simulink model "advisor_ess_options"  (Simulink 2.20)
settings: Solver=ode1  StartTime=0.0  StopTime=500  FixedStep=1  RelTol=1e-3
values from neighbouring files (symbols this model uses):
  amb_tmp = vinf.test.ambtmp    [RW_execute.m]
  cyc_mph = [time speed]    [DataCompareFigControl.m]    (also in J17_FUDS.m = [time_vec speed_vec]; J17_HFEDS.m = [time_vec speed_vec]; J17_SC03.m = [time_vec speed_vec]; J17_UDDS.m = [time_vec speed_vec])
  ess_init_soc = vinf.test.ess_init_soc.FUDS    [J17_FUDS.m]    (also in J17_HFEDS.m = vinf.test.ess_init_soc.HWFET; J17_SC03.m = vinf.test.ess_init_soc.SC03; J17_UDDS.m = vinf.test.ess_init_soc.UDDS; J17_US06.m = vinf.test.ess_init_soc.US06)
undefined symbols (not defined in the file or in its folder): air_cp, enable_stop, ess_coulombic_eff, ess_max_ah_cap, ess_max_p, ess_max_p_soc, ess_max_volts, ess_min_volts, ess_MMi, ess_MMo, ess_mod_airflow, ess_mod_cp, ess_mod_init_tmp, ess_module_mass, ess_module_num, ess_on, ess_set_tmp, ess_th_calc, ess_th_res_off, ess_th_res_on, ess_tmp, fund_byu, fund_byuop, mc_min_volts, t_soc
(part 1 of 2)
settings Model: ConsistencyChecking=off  RTWPlaceOutputsASAP=off

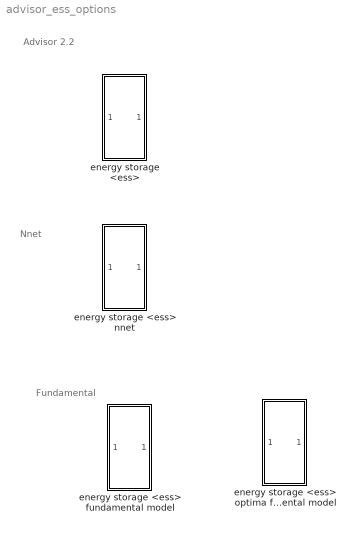
== system advisor_ess_options ==
  note: Nnet
  note: Fundamental
  note: Advisor 2.2
  energy storage <ess> : Subsystem
  energy storage <ess> nnet : Subsystem
  energy storage <ess> fundamental model : Subsystem
  energy storage <ess> optima fundamental model : Subsystem

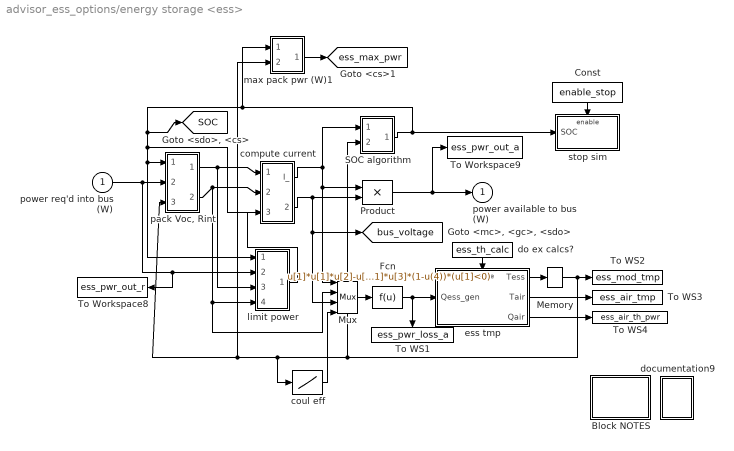
== system advisor_ess_options/energy storage <ess> ==
  power req'd into bus (W) : Inport  Port=1  PortWidth=-1  SampleTime=-1
  Block NOTES : Subsystem
      mask Display: disp('Block\nNOTES')
  Const : Constant  Orientation=down  Value=enable_stop
  Fcn : Fcn  Expr=u[1]*u[1]*u[2]-u[1]*u[3]*(1-u(4))*(u[1]<0)
  Memory : Memory  X0=amb_tmp  InheritSampleTime=off
  Mux : Mux  Inputs=4
  Product : Product  Inputs=2
  SOC algorithm : Subsystem
  To WS1 : ToWorkspace  VariableName=ess_pwr_loss_a  SampleTime=0
      settings: Orientation=down
  To WS2 : ToWorkspace  VariableName=ess_mod_tmp  SampleTime=0
  To WS3 : ToWorkspace  VariableName=ess_air_tmp  SampleTime=0
  To WS4 : ToWorkspace  VariableName=ess_air_th_pwr  SampleTime=0
  To Workspace8 : ToWorkspace  VariableName=ess_pwr_out_r  SampleTime=-1
  To Workspace9 : ToWorkspace  VariableName=ess_pwr_out_a  SampleTime=-1
  compute current : Subsystem
  coul eff : Lookup  InputValues=ess_tmp  OutputValues=ess_coulombic_eff
  do ex calcs? : Constant  Orientation=down  Value=ess_th_calc
  documentation9 : Subsystem
      settings: OpenFcn=web(['file:\\\' which('energy_storage.htm')]);
      mask Display: image(imread('doc_man.jpg'))
  ess tmp : Subsystem
  limit power : Subsystem
  max pack pwr (W)1 : Subsystem
  "pack Voc, Rint" : Subsystem
  stop sim : Subsystem
  power available to bus (W) : Outport  Port=1  InitialOutput=0
  tag scope: SOC=global, bus_voltage=global, ess_max_pwr=global
  wires:
  Memory/1 -> max pack pwr (W)1/2(ess_mod_tmp), "pack Voc, Rint"/3(mod tmp   (C)), coul eff/1, SOC algorithm/2(tmp (C)), To WS2/1
  max pack pwr (W)1/1(max ess discharge pwr) -> [ess_max_pwr]
  coul eff/1 -> Mux/4
  ess tmp/1(Tess) -> Memory/1
  ess tmp/3(Qair) -> To WS4/1
  ess tmp/2(Tair) -> To WS3/1
  limit power/1("Pbty, limited") -> compute current/3(limited output power (W))
  "pack Voc, Rint"/1(pack open- circuit voltage) -> limit power/3(Voc), compute current/1(Voc)
  "pack Voc, Rint"/2(pack resistance) -> Mux/2, limit power/4(Rint), compute current/2(Rint)
  Const/1 -> stop sim/Enable
  SOC algorithm/1(SOC1) -> max pack pwr (W)1/1(SOC), limit power/1(SOC), "pack Voc, Rint"/1(SOC (prev)), [SOC], stop sim/1(SOC)
  do ex calcs?/1 -> ess tmp/Enable
  Fcn/1 -> ess tmp/1(Qess_gen), To WS1/1
  Product/1 -> power available to bus (W)/1, To Workspace9/1
  compute current/1(I_) -> Mux/1, Product/1, SOC algorithm/1((A))
  power req'd into bus (W)/1 -> "pack Voc, Rint"/2(req'd battery power (W)), limit power/2(Pbty), To Workspace8/1
  Mux/1 -> Fcn/1
  compute current/2(V_) -> [bus_voltage], Mux/3, Product/2

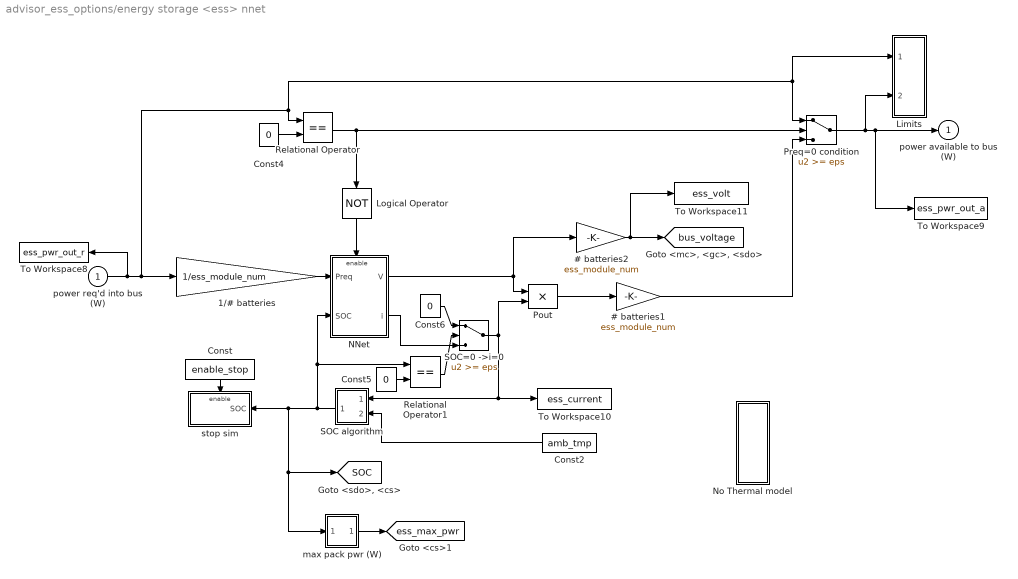
== system advisor_ess_options/energy storage <ess> nnet ==
  power req'd into bus (W) : Inport  Port=1  PortWidth=-1  SampleTime=-1
  # batteries1 : Gain  Gain=ess_module_num
  # batteries2 : Gain  Gain=ess_module_num
  1/# batteries : Gain  Gain=1/ess_module_num
  Const : Constant  Orientation=down  Value=enable_stop
  Const2 : Constant  Orientation=left  Value=amb_tmp
  Const4 : Constant  Value=0
  Const5 : Constant  Value=0
  Const6 : Constant  Value=0
  Limits : Subsystem
  Logical Operator : Logic  Orientation=down  Operator=NOT  Inputs=1
  NNet : Subsystem
  No Thermal model : Subsystem
  Pout : Product  Inputs=2
  Preq=0 condition : Switch  Threshold=eps
  Relational Operator : RelationalOperator  Operator===
  Relational Operator1 : RelationalOperator  Operator===
  SOC algorithm : Subsystem  Orientation=left
  SOC=0 ->i=0 : Switch  Threshold=eps
  To Workspace10 : ToWorkspace  VariableName=ess_current  SampleTime=-1
  To Workspace11 : ToWorkspace  VariableName=ess_volt  SampleTime=-1
  To Workspace8 : ToWorkspace  VariableName=ess_pwr_out_r  SampleTime=-1
  To Workspace9 : ToWorkspace  VariableName=ess_pwr_out_a  SampleTime=-1
  max pack pwr (W) : Subsystem
  stop sim : Subsystem  Orientation=left
  power available to bus (W) : Outport  Port=1  InitialOutput=0
  tag scope: SOC=global, bus_voltage=global, ess_max_pwr=global
  wires:
  Const/1 -> stop sim/Enable
  SOC algorithm/1(SOC1) -> stop sim/1(SOC), [SOC], max pack pwr (W)/1(SOC), NNet/2(SOC), Relational Operator1/1
  power req'd into bus (W)/1 -> To Workspace8/1, 1/# batteries/1, Relational Operator/1, Preq=0 condition/1, Limits/1(power req)
  1/# batteries/1 -> NNet/1(Preq)
  Const4/1 -> Relational Operator/2
  Logical Operator/1 -> NNet/Enable
  Relational Operator/1 -> Preq=0 condition/2, Logical Operator/1
  max pack pwr (W)/1(ess discharge pwr) -> [ess_max_pwr]
  Pout/1 -> # batteries1/1
  NNet/1(V) -> Pout/1, # batteries2/1
  # batteries2/1 -> [bus_voltage], To Workspace11/1
  # batteries1/1 -> Preq=0 condition/3
  Preq=0 condition/1 -> power available to bus (W)/1, To Workspace9/1, Limits/2(power  available from battery)
  Const2/1 -> SOC algorithm/2(tmp (C))
  Const6/1 -> SOC=0 ->i=0/1
  NNet/2(i) -> SOC=0 ->i=0/3
  Const5/1 -> Relational Operator1/2
  Relational Operator1/1 -> SOC=0 ->i=0/2
  SOC=0 ->i=0/1 -> SOC algorithm/1((A)), To Workspace10/1, Pout/2

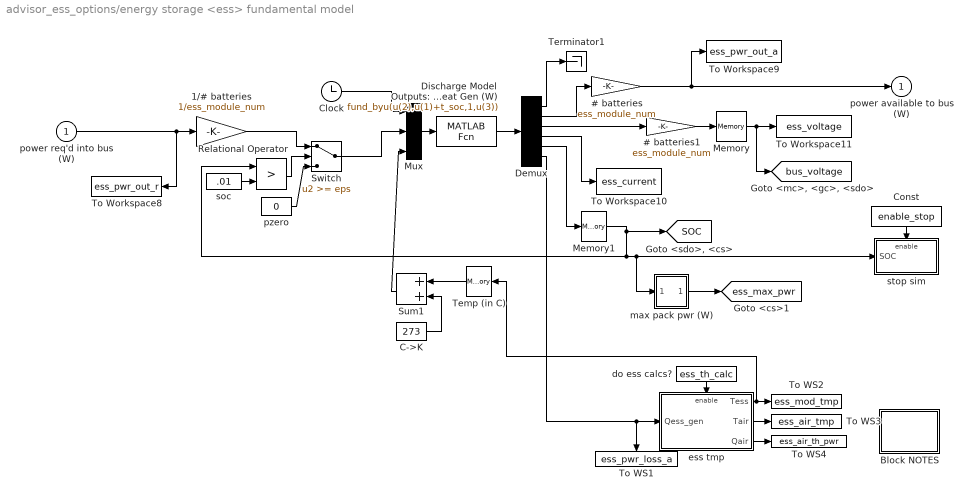
== system advisor_ess_options/energy storage <ess> fundamental model ==
  power req'd into bus (W) : Inport  Port=1  PortWidth=-1  SampleTime=-1
  # batteries : Gain  Gain=ess_module_num
  # batteries1 : Gain  Gain=ess_module_num
  1/# batteries : Gain  Gain=1/ess_module_num
  Block NOTES : Subsystem
      mask Display: disp('Block\nNOTES')
  C->K : Constant  Value=273
  Clock : Clock
  Const : Constant  Orientation=down  Value=enable_stop
  Demux : Demux  Outputs=6
  Discharge Model Outputs: Preq(W) Pavail (W) Voltage (V) Current (A) SOC Heat Gen (W) : MATLABFcn  MATLABFcn=fund_byu(u(2),u(1)+t_soc,1,u(3))  OutputWidth=-1
  Memory : Memory  X0=12*ess_module_num  InheritSampleTime=off
  Memory1 : Memory  X0=ess_init_soc  InheritSampleTime=off
  Mux : Mux  Inputs=3
  Relational Operator : RelationalOperator  Operator=>
  Sum1 : Sum  Orientation=left  Inputs=++
  Switch : Switch  Threshold=eps
  Temp (in C) : Memory  Orientation=left  X0=amb_tmp  InheritSampleTime=off
  Terminator1 : Terminator
  To WS1 : ToWorkspace  VariableName=ess_pwr_loss_a  SampleTime=0
      settings: Orientation=down  Buffer=50000
  To WS2 : ToWorkspace  VariableName=ess_mod_tmp  SampleTime=0
      settings: Buffer=50000
  To WS3 : ToWorkspace  VariableName=ess_air_tmp  SampleTime=0
      settings: Buffer=50000
  To WS4 : ToWorkspace  VariableName=ess_air_th_pwr  SampleTime=0
      settings: Buffer=50000
  To Workspace10 : ToWorkspace  VariableName=ess_current  SampleTime=-1
  To Workspace11 : ToWorkspace  VariableName=ess_voltage  SampleTime=-1
  To Workspace8 : ToWorkspace  VariableName=ess_pwr_out_r  SampleTime=-1
  To Workspace9 : ToWorkspace  VariableName=ess_pwr_out_a  SampleTime=-1
  do ess calcs? : Constant  Orientation=down  Value=ess_th_calc
  ess tmp : Subsystem
  max pack pwr (W) : Subsystem
  pzero : Constant  Value=0
  soc : Constant  Value=.01
  stop sim : Subsystem
  power available to bus (W) : Outport  Port=1  InitialOutput=0
  tag scope: SOC=global, bus_voltage=global, ess_max_pwr=global
  wires:
  Mux/1 -> Discharge Model Outputs: Preq(W) Pavail (W) Voltage (V) Current (A) SOC Heat Gen (W)/1
  Discharge Model Outputs: Preq(W) Pavail (W) Voltage (V) Current (A) SOC Heat Gen (W)/1 -> Demux/1
  Demux/5 -> Memory1/1
  Demux/4 -> To Workspace10/1
  Demux/2 -> # batteries/1
  Clock/1 -> Mux/1
  power req'd into bus (W)/1 -> To Workspace8/1, 1/# batteries/1
  pzero/1 -> Switch/3
  Relational Operator/1 -> Switch/2
  soc/1 -> Relational Operator/2
  1/# batteries/1 -> Switch/1
  Switch/1 -> Mux/2
  Demux/1 -> Terminator1/1
  # batteries/1 -> To Workspace9/1, power available to bus (W)/1
  # batteries1/1 -> Memory/1
  Demux/3 -> # batteries1/1
  Memory/1 -> To Workspace11/1, [bus_voltage]
  Memory1/1 -> Relational Operator/1, stop sim/1(SOC), max pack pwr (W)/1(SOC), [SOC]
  Temp (in C)/1 -> Sum1/1
  C->K/1 -> Sum1/2
  Sum1/1 -> Mux/3
  Const/1 -> stop sim/Enable
  max pack pwr (W)/1(ess discharge pwr) -> [ess_max_pwr]
  Demux/6 -> ess tmp/1(Qess_gen), To WS1/1
  do ess calcs?/1 -> ess tmp/Enable
  ess tmp/2(Tair) -> To WS3/1
  ess tmp/3(Qair) -> To WS4/1
  ess tmp/1(Tess) -> To WS2/1, Temp (in C)/1

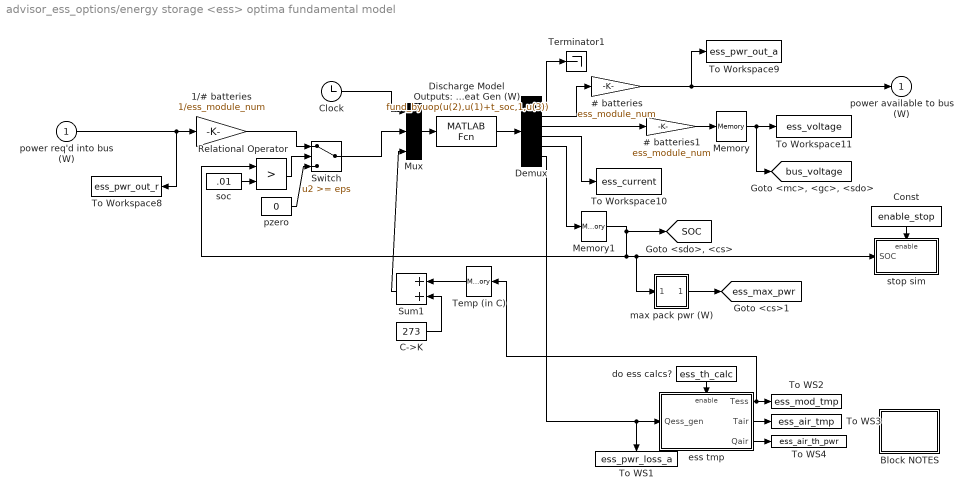
== system advisor_ess_options/energy storage <ess> optima fundamental model ==
  power req'd into bus (W) : Inport  Port=1  PortWidth=-1  SampleTime=-1
  # batteries : Gain  Gain=ess_module_num
  # batteries1 : Gain  Gain=ess_module_num
  1/# batteries : Gain  Gain=1/ess_module_num
  Block NOTES : Subsystem
      mask Display: disp('Block\nNOTES')
  C->K : Constant  Value=273
  Clock : Clock
  Const : Constant  Orientation=down  Value=enable_stop
  Demux : Demux  Outputs=6
  Discharge Model Outputs: Preq(W) Pavail (W) Voltage (V) Current (A) SOC Heat Gen (W) : MATLABFcn  MATLABFcn=fund_byuop(u(2),u(1)+t_soc,1,u(3))  OutputWidth=-1
  Memory : Memory  X0=12*ess_module_num  InheritSampleTime=off
  Memory1 : Memory  X0=ess_init_soc  InheritSampleTime=off
  Mux : Mux  Inputs=3
  Relational Operator : RelationalOperator  Operator=>
  Sum1 : Sum  Orientation=left  Inputs=++
  Switch : Switch  Threshold=eps
  Temp (in C) : Memory  Orientation=left  X0=amb_tmp  InheritSampleTime=off
  Terminator1 : Terminator
  To WS1 : ToWorkspace  VariableName=ess_pwr_loss_a  SampleTime=0
      settings: Orientation=down  Buffer=50000
  To WS2 : ToWorkspace  VariableName=ess_mod_tmp  SampleTime=0
      settings: Buffer=50000
  To WS3 : ToWorkspace  VariableName=ess_air_tmp  SampleTime=0
      settings: Buffer=50000
  To WS4 : ToWorkspace  VariableName=ess_air_th_pwr  SampleTime=0
      settings: Buffer=50000
  To Workspace10 : ToWorkspace  VariableName=ess_current  SampleTime=-1
  To Workspace11 : ToWorkspace  VariableName=ess_voltage  SampleTime=-1
  To Workspace8 : ToWorkspace  VariableName=ess_pwr_out_r  SampleTime=-1
  To Workspace9 : ToWorkspace  VariableName=ess_pwr_out_a  SampleTime=-1
  do ess calcs? : Constant  Orientation=down  Value=ess_th_calc
  ess tmp : Subsystem
  max pack pwr (W) : Subsystem
  pzero : Constant  Value=0
  soc : Constant  Value=.01
  stop sim : Subsystem
  power available to bus (W) : Outport  Port=1  InitialOutput=0
  tag scope: SOC=global, bus_voltage=global, ess_max_pwr=global
  wires:
  Mux/1 -> Discharge Model Outputs: Preq(W) Pavail (W) Voltage (V) Current (A) SOC Heat Gen (W)/1
  Discharge Model Outputs: Preq(W) Pavail (W) Voltage (V) Current (A) SOC Heat Gen (W)/1 -> Demux/1
  Demux/5 -> Memory1/1
  Demux/4 -> To Workspace10/1
  Demux/2 -> # batteries/1
  Clock/1 -> Mux/1
  power req'd into bus (W)/1 -> To Workspace8/1, 1/# batteries/1
  pzero/1 -> Switch/3
  Relational Operator/1 -> Switch/2
  soc/1 -> Relational Operator/2
  1/# batteries/1 -> Switch/1
  Switch/1 -> Mux/2
  Demux/1 -> Terminator1/1
  # batteries/1 -> To Workspace9/1, power available to bus (W)/1
  # batteries1/1 -> Memory/1
  Demux/3 -> # batteries1/1
  Memory/1 -> To Workspace11/1, [bus_voltage]
  Memory1/1 -> Relational Operator/1, stop sim/1(SOC), max pack pwr (W)/1(SOC), [SOC]
  Temp (in C)/1 -> Sum1/1
  C->K/1 -> Sum1/2
  Sum1/1 -> Mux/3
  Const/1 -> stop sim/Enable
  max pack pwr (W)/1(ess discharge pwr) -> [ess_max_pwr]
  Demux/6 -> ess tmp/1(Qess_gen), To WS1/1
  do ess calcs?/1 -> ess tmp/Enable
  ess tmp/2(Tair) -> To WS3/1
  ess tmp/3(Qair) -> To WS4/1
  ess tmp/1(Tess) -> To WS2/1, Temp (in C)/1

== system advisor_ess_options/energy storage <ess>/Block NOTES ==
  note: This block models the energy storage system as an SOC-dependent voltage
      | in series with an SOC- and current direction-dependent internal resistance.
      | SOC is computed assuming that A-h capacity is constant, but limited
      | such that a minimum voltage is never exceeded (replacing the
      | previous Peukert relationship which underpredicted battery capacity).
      |
      | Discharge power is limited here so as not to bring the bus (battery pack) voltage below
      | the minimum controller voltage or the minimum battery voltage and so as to allow
      | the solution of the quadratic eq'n for discharge current.
      |
      | Charge current is limited to ensure the voltage does not exceed a maximum
      | voltage
      |
      | Positive current is discharge current in the convention used here.
      | Power loss is computed as I*R+losses due to Coulombic (in)efficiency.
      |
      | Thermal modeling of the battery performance is modeled in the
      | OCV, Rint, and capacity.

== system advisor_ess_options/energy storage <ess>/SOC algorithm ==
  note: SOC=(Max Ah capacity-Ah used)/Max Ah capacity
  (A) : Inport  Port=1  PortWidth=-1  SampleTime=-1
  tmp (C) : Inport  Port=2  PortWidth=-1  SampleTime=-1
  (sec->hrs) : Gain  Gain=1/3600
  0 <= SOC <= 1 : Saturate  UpperLimit=1  LowerLimit=0
  A-h remaining : Sum  Inputs=-+
  Ah used : Integrator  ExternalReset=none  InitialConditionSource=external  InitialCondition=(1-ess_init_soc)*ess_max_ah_cap  LimitOutput=off  UpperSaturationLimit=inf  LowerSaturationLimit=-inf  ShowSaturationPort=off  ShowStatePort=off  AbsoluteTolerance=auto
  Fcn : Fcn  Expr=1/u
  Fcn1 : Fcn  Expr=(1-ess_init_soc)*u
  SOC : Product  Inputs=2
  Switch : Switch  Threshold=0
  adjusted A : Product  Inputs=2
  coul eff : Lookup  InputValues=ess_tmp  OutputValues=ess_coulombic_eff
  max cap : Lookup  InputValues=ess_tmp  OutputValues=ess_max_ah_cap
  SOC1 : Outport  Port=1  InitialOutput=0
  wires:
  Fcn1/1 -> Ah used/2
  max cap/1 -> Fcn1/1, Fcn/1, A-h remaining/2
  adjusted A/1 -> Switch/3
  coul eff/1 -> adjusted A/2
  tmp (C)/1 -> coul eff/1, max cap/1
  0 <= SOC <= 1/1 -> SOC1/1
  A-h remaining/1 -> SOC/1
  SOC/1 -> 0 <= SOC <= 1/1
  Fcn/1 -> SOC/2
  Ah used/1 -> A-h remaining/1
  (sec->hrs)/1 -> Ah used/1
  Switch/1 -> (sec->hrs)/1
  (A)/1 -> adjusted A/1, Switch/1, Switch/2

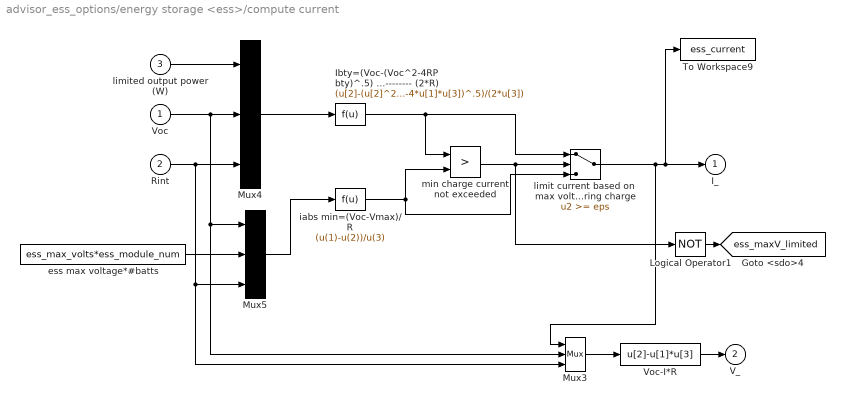
== system advisor_ess_options/energy storage <ess>/compute current ==
  Voc : Inport  Port=1  PortWidth=-1  SampleTime=-1
  Rint : Inport  Port=2  PortWidth=-1  SampleTime=-1
  limited output power (W) : Inport  Port=3  PortWidth=-1  SampleTime=-1
  Ibty=(Voc-(Voc^2-4RPbty)^.5)        ----------------------------- (2*R) : Fcn  Expr=(u[2]-(u[2]^2-4*u[1]*u[3])^.5)/(2*u[3])
  Logical Operator1 : Logic  Operator=NOT  Inputs=1
  Mux3 : Mux  Inputs=3
  Mux4 : Mux  Inputs=3
  Mux5 : Mux  Inputs=3
  To Workspace9 : ToWorkspace  VariableName=ess_current  SampleTime=-1
  Voc-I*R : Fcn  Expr=u[2]-u[1]*u[3]
  ess max voltage*#batts : Constant  Value=ess_max_volts*ess_module_num
  iabs min=(Voc-Vmax)/R : Fcn  Expr=(u(1)-u(2))/u(3)
  limit current based on  max voltage during charge : Switch  Threshold=eps
  min charge current not exceeded : RelationalOperator  Operator=>
  I_ : Outport  Port=1  InitialOutput=0
  V_ : Outport  Port=2  InitialOutput=0
  tag scope: ess_maxV_limited=global
  wires:
  Logical Operator1/1 -> [ess_maxV_limited]
  ess max voltage*#batts/1 -> Mux5/2
  Mux5/1 -> iabs min=(Voc-Vmax)/R/1
  Mux4/1 -> Ibty=(Voc-(Voc^2-4RPbty)^.5)        ----------------------------- (2*R)/1
  Voc-I*R/1 -> V_/1
  Mux3/1 -> Voc-I*R/1
  min charge current not exceeded/1 -> Logical Operator1/1, limit current based on  max voltage during charge/2
  limit current based on  max voltage during charge/1 -> Mux3/1, To Workspace9/1, I_/1
  iabs min=(Voc-Vmax)/R/1 -> limit current based on  max voltage during charge/3, min charge current not exceeded/2
  Ibty=(Voc-(Voc^2-4RPbty)^.5)        ----------------------------- (2*R)/1 -> limit current based on  max voltage during charge/1, min charge current not exceeded/1
  Rint/1 -> Mux5/3, Mux3/3, Mux4/3
  Voc/1 -> Mux5/1, Mux3/2, Mux4/2
  limited output power (W)/1 -> Mux4/1

== system advisor_ess_options/energy storage <ess>/documentation9 ==

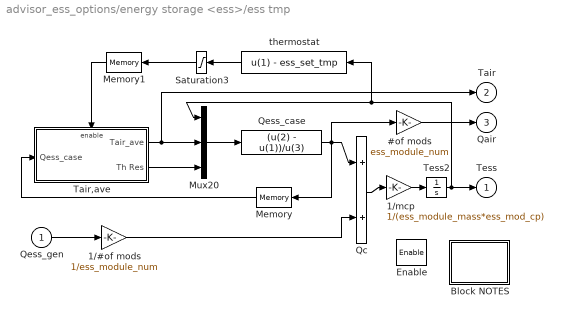
== system advisor_ess_options/energy storage <ess>/ess tmp ==
  Qess_gen : Inport  Port=1  PortWidth=-1  SampleTime=-1
  Enable : EnablePort  StatesWhenEnabling=reset
  #of mods : Gain  Gain=ess_module_num
  1/#of mods : Gain  Gain=1/ess_module_num
  1/mcp : Gain  Gain=1/(ess_module_mass*ess_mod_cp)
  Block NOTES : Subsystem
      mask Display: disp('Block\nNOTES')
  Memory : Memory  Orientation=left  X0=cyc_mph(1,2)*.447  InheritSampleTime=off
  Memory1 : Memory  Orientation=left  X0=cyc_mph(1,2)*.447  InheritSampleTime=off
  Mux20 : Mux  Inputs=3
  Qc : Sum  Inputs=++
  Qess_case : Fcn  Expr=(u(2) - u(1))/u(3)
  Saturation3 : Saturate  Orientation=left  UpperLimit=1  LowerLimit=0
  Tair,ave : Subsystem
  Tess2 : Integrator  ExternalReset=none  InitialConditionSource=internal  InitialCondition=ess_mod_init_tmp  LimitOutput=off  UpperSaturationLimit=inf  LowerSaturationLimit=-inf  ShowSaturationPort=off  ShowStatePort=off  AbsoluteTolerance=auto
  thermostat : Fcn  Orientation=left  Expr=u(1) - ess_set_tmp
  Tess : Outport  Port=1  InitialOutput=0
  Tair : Outport  Port=2
  Qair : Outport  Port=3  OutputWhenDisabled=reset  InitialOutput=0
  wires:
  Tair,ave/1(Tair_ave) -> Tair/1, Mux20/2
  Tair,ave/2(Th Res) -> Mux20/3
  Mux20/1 -> Qess_case/1
  #of mods/1 -> Qair/1
  Memory/1 -> Tair,ave/1(Qess_case)
  Memory1/1 -> Tair,ave/Enable
  Saturation3/1 -> Memory1/1
  thermostat/1 -> Saturation3/1
  1/#of mods/1 -> Qc/2
  Qess_gen/1 -> 1/#of mods/1
  Tess2/1 -> thermostat/1, Mux20/1, Tess/1
  1/mcp/1 -> Tess2/1
  Qess_case/1 -> #of mods/1, Memory/1, Qc/1
  Qc/1 -> 1/mcp/1

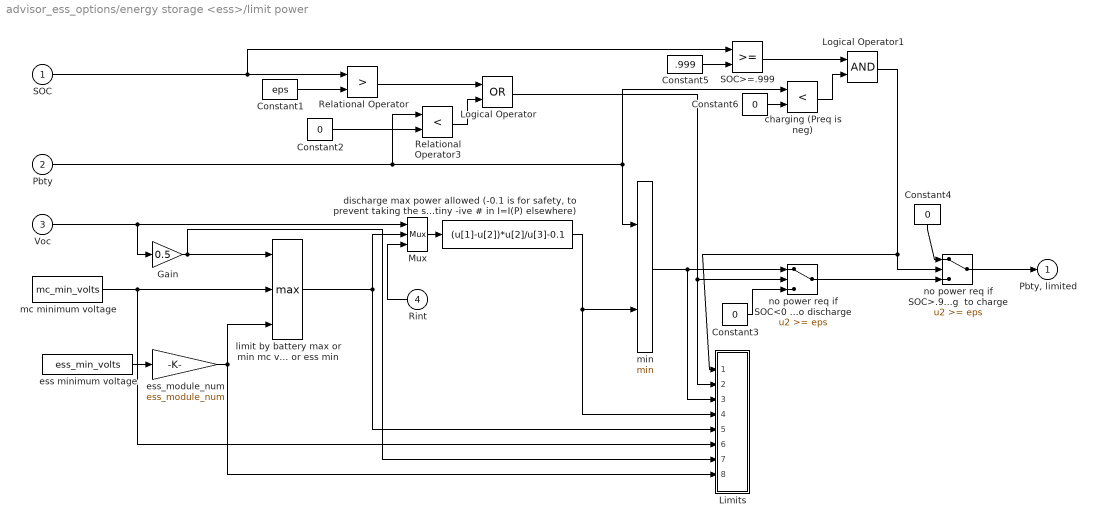
== system advisor_ess_options/energy storage <ess>/limit power ==
  SOC : Inport  Port=1  PortWidth=-1  SampleTime=-1
  Pbty : Inport  Port=2  PortWidth=-1  SampleTime=-1
  Voc : Inport  Port=3  PortWidth=-1  SampleTime=-1
  Rint : Inport  Orientation=left  Port=4  PortWidth=-1  SampleTime=-1
  Constant1 : Constant  Value=eps
  Constant2 : Constant  Value=0
  Constant3 : Constant  Value=0
  Constant4 : Constant  Orientation=down  Value=0
  Constant5 : Constant  Value=.999
  Constant6 : Constant  Value=0
  Gain : Gain  Gain=0.5
  Limits : Subsystem
  Logical Operator : Logic  Operator=OR  Inputs=2
  Logical Operator1 : Logic  Operator=AND  Inputs=2
  Mux : Mux  Inputs=3
  Relational Operator : RelationalOperator  Operator=>
  Relational Operator3 : RelationalOperator  Operator=<
  SOC>=.999 : RelationalOperator  Operator=>=
  charging (Preq is neg) : RelationalOperator  Operator=<
  "discharge max power allowed (-0.1 is for safety, to prevent taking the square of a tiny -ive # in I=I(P) elsewhere)" : Fcn  Expr=(u[1]-u[2])*u[2]/u[3]-0.1
  ess minimum voltage : Constant  Value=ess_min_volts
  ess_module_num : Gain  Gain=ess_module_num
  limit by battery max or min mc voltage or ess min : MinMax  Function=max  Inputs=3
  mc minimum voltage : Constant  Value=mc_min_volts
  min : MinMax  Function=min  Inputs=2
  no power req if SOC<0 and trying  to discharge : Switch  Threshold=eps
  no power req if SOC>.999 and trying  to charge : Switch  Threshold=eps
  "Pbty, limited" : Outport  Port=1  InitialOutput=0
  wires:
  Logical Operator1/1 -> Limits/1(SOC  high limited), no power req if SOC>.999 and trying  to charge/2
  no power req if SOC>.999 and trying  to charge/1 -> "Pbty, limited"/1
  no power req if SOC<0 and trying  to discharge/1 -> no power req if SOC>.999 and trying  to charge/3
  Constant4/1 -> no power req if SOC>.999 and trying  to charge/1
  Constant5/1 -> SOC>=.999/2
  charging (Preq is neg)/1 -> Logical Operator1/2
  Constant6/1 -> charging (Preq is neg)/2
  SOC>=.999/1 -> Logical Operator1/1
  SOC/1 -> SOC>=.999/1, Relational Operator/1
  ess_module_num/1 -> Limits/8(V ess_min_volts), limit by battery max or min mc voltage or ess min/3
  ess minimum voltage/1 -> ess_module_num/1
  Gain/1 -> Limits/7(V battery (.5Voc)), limit by battery max or min mc voltage or ess min/1
  Rint/1 -> Mux/3
  mc minimum voltage/1 -> Limits/6(V mc_min_volts), limit by battery max or min mc voltage or ess min/2
  "discharge max power allowed (-0.1 is for safety, to prevent taking the square of a tiny -ive # in I=I(P) elsewhere)"/1 -> min/2, Limits/4(power bat limited)
  limit by battery max or min mc voltage or ess min/1 -> Limits/5(V used), Mux/2
  Mux/1 -> "discharge max power allowed (-0.1 is for safety, to prevent taking the square of a tiny -ive # in I=I(P) elsewhere)"/1
  min/1 -> Limits/3(power req), no power req if SOC<0 and trying  to discharge/1
  Voc/1 -> Gain/1, Mux/1
  Logical Operator/1 -> Limits/2(not SOC  low limited), no power req if SOC<0 and trying  to discharge/2
  Constant3/1 -> no power req if SOC<0 and trying  to discharge/3
  Relational Operator3/1 -> Logical Operator/2
  Constant2/1 -> Relational Operator3/2
  Pbty/1 -> charging (Preq is neg)/1, min/1, Relational Operator3/1
  Relational Operator/1 -> Logical Operator/1
  Constant1/1 -> Relational Operator/2

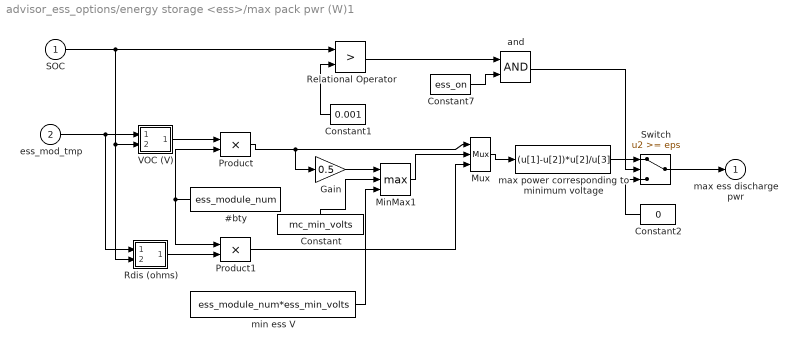
== system advisor_ess_options/energy storage <ess>/max pack pwr (W)1 ==
  SOC : Inport  Port=1  PortWidth=-1  SampleTime=-1
  ess_mod_tmp : Inport  Port=2  PortWidth=-1  SampleTime=-1
  #bty : Constant  Orientation=left  Value=ess_module_num
  Constant : Constant  Orientation=up  Value=mc_min_volts
  Constant1 : Constant  Orientation=left  Value=0.001
  Constant2 : Constant  Orientation=left  Value=0
  Constant7 : Constant  Value=ess_on
  Gain : Gain  Gain=0.5
  MinMax1 : MinMax  Function=max  Inputs=3
  Mux : Mux  Inputs=3
  Product : Product  Inputs=2
  Product1 : Product  Inputs=2
  Rdis (ohms) : Subsystem  mask(2-D Table Lookup){@1=ess_tmp, @2=ess_soc, @3=ess_r_dis}
      mask prompts: @1 "X Index"; @2 "Y Index"; @3 "Table"
      mask help:
      | Two Dimensional Table Lookup
      | The first input corresponds to X Index and the second input corresponds to the Y Index
      mask init:
      | xindex=@1; yindex=@2; table=@3; sftab2chk(xindex,yindex,table);
      mask Help: This block returns a linearly interpolated intersection from the table using the X index (which corresponds to the rows of the table) and the Y index (which corresponds to the columns of the table).  Extrapolation is used.
      mask Display: plot(-10,-10,110,110,[90,50,10],[90,40,30],[90,50,10],[50,26,20],[90,50,10],[22,13,10])
  Relational Operator : RelationalOperator  Operator=>
  Switch : Switch  Threshold=eps
  VOC (V) : Subsystem  mask(2-D Table Lookup){@1=ess_tmp, @2=ess_soc, @3=ess_voc}
      mask prompts: @1 "X Index"; @2 "Y Index"; @3 "Table"
      mask help:
      | Two Dimensional Table Lookup
      | The first input corresponds to X Index and the second input corresponds to the Y Index
      mask init:
      | xindex=@1; yindex=@2; table=@3; sftab2chk(xindex,yindex,table);
      mask Help: This block returns a linearly interpolated intersection from the table using the X index (which corresponds to the rows of the table) and the Y index (which corresponds to the columns of the table).  Extrapolation is used.
      mask Display: plot(-10,-10,110,110,[90,50,10],[90,40,30],[90,50,10],[50,26,20],[90,50,10],[22,13,10])
  and : Logic  Operator=AND  Inputs=2
  max power corresponding to minimum voltage : Fcn  Expr=(u[1]-u[2])*u[2]/u[3]
  min ess V : Constant  Value=ess_module_num*ess_min_volts
  max ess discharge pwr : Outport  Port=1  InitialOutput=0
  wires:
  Switch/1 -> max ess discharge pwr/1
  SOC/1 -> VOC (V)/2(y0), Rdis (ohms)/2(y0), Relational Operator/1
  Constant2/1 -> Switch/3
  max power corresponding to minimum voltage/1 -> Switch/1
  #bty/1 -> Product1/1, Product/2
  Rdis (ohms)/1(table out) -> Product1/2
  VOC (V)/1(table out) -> Product/1
  Product1/1 -> Mux/3
  Product/1 -> Gain/1, Mux/1
  MinMax1/1 -> Mux/2
  Gain/1 -> MinMax1/1
  Mux/1 -> max power corresponding to minimum voltage/1
  Constant/1 -> MinMax1/2
  Constant1/1 -> Relational Operator/2
  ess_mod_tmp/1 -> VOC (V)/1(x0), Rdis (ohms)/1(x0)
  min ess V/1 -> MinMax1/3
  and/1 -> Switch/2
  Relational Operator/1 -> and/1
  Constant7/1 -> and/2

== system advisor_ess_options/energy storage <ess>/pack Voc, Rint ==
  SOC (prev) : Inport  Port=1  PortWidth=-1  SampleTime=-1
  req'd battery power (W) : Inport  Port=2  PortWidth=-1  SampleTime=-1
  mod tmp   (C) : Inport  Port=3  PortWidth=-1  SampleTime=-1
  #bty : Constant  Value=ess_module_num
  Product : Product  Inputs=2
  Product1 : Product  Inputs=2
  Rchg (ohms) : Subsystem  mask(2-D Table Lookup){@1=ess_tmp, @2=ess_soc, @3=ess_r_chg}
      mask prompts: @1 "X Index"; @2 "Y Index"; @3 "Table"
      mask help:
      | Two Dimensional Table Lookup
      | The first input corresponds to X Index and the second input corresponds to the Y Index
      mask init:
      | xindex=@1; yindex=@2; table=@3; sftab2chk(xindex,yindex,table);
      mask Help: This block returns a linearly interpolated intersection from the table using the X index (which corresponds to the rows of the table) and the Y index (which corresponds to the columns of the table).  Extrapolation is used.
      mask Display: plot(-10,-10,110,110,[90,50,10],[90,40,30],[90,50,10],[50,26,20],[90,50,10],[22,13,10])
  Rdis (ohms) : Subsystem  mask(2-D Table Lookup){@1=ess_tmp, @2=ess_soc, @3=ess_r_dis}
      mask prompts: @1 "X Index"; @2 "Y Index"; @3 "Table"
      mask help:
      | Two Dimensional Table Lookup
      | The first input corresponds to X Index and the second input corresponds to the Y Index
      mask init:
      | xindex=@1; yindex=@2; table=@3; sftab2chk(xindex,yindex,table);
      mask Help: This block returns a linearly interpolated intersection from the table using the X index (which corresponds to the rows of the table) and the Y index (which corresponds to the columns of the table).  Extrapolation is used.
      mask Display: plot(-10,-10,110,110,[90,50,10],[90,40,30],[90,50,10],[50,26,20],[90,50,10],[22,13,10])
  Switch : Switch  Threshold=0
  VOC (V) : Subsystem  mask(2-D Table Lookup){@1=ess_tmp, @2=ess_soc, @3=ess_voc}
      mask prompts: @1 "X Index"; @2 "Y Index"; @3 "Table"
      mask help:
      | Two Dimensional Table Lookup
      | The first input corresponds to X Index and the second input corresponds to the Y Index
      mask init:
      | xindex=@1; yindex=@2; table=@3; sftab2chk(xindex,yindex,table);
      mask Help: This block returns a linearly interpolated intersection from the table using the X index (which corresponds to the rows of the table) and the Y index (which corresponds to the columns of the table).  Extrapolation is used.
      mask Display: plot(-10,-10,110,110,[90,50,10],[90,40,30],[90,50,10],[50,26,20],[90,50,10],[22,13,10])
  pack open- circuit voltage : Outport  Port=1  InitialOutput=0
  pack resistance : Outport  Port=2  InitialOutput=0
  wires:
  mod tmp   (C)/1 -> Rchg (ohms)/1(x0), Rdis (ohms)/1(x0), VOC (V)/1(x0)
  SOC (prev)/1 -> Rchg (ohms)/2(y0), Rdis (ohms)/2(y0), VOC (V)/2(y0)
  Switch/1 -> Product1/2
  req'd battery power (W)/1 -> Switch/2
  Rdis (ohms)/1(table out) -> Switch/1
  Rchg (ohms)/1(table out) -> Switch/3
  VOC (V)/1(table out) -> Product/1
  #bty/1 -> Product/2, Product1/1
  Product1/1 -> pack resistance/1
  Product/1 -> pack open- circuit voltage/1

== system advisor_ess_options/energy storage <ess>/stop sim ==
  SOC : Inport  Port=1  PortWidth=-1  SampleTime=-1
  Enable : EnablePort
  Const : Constant  Orientation=up  Value=.001
  Relational Operator : RelationalOperator  Operator=<
  Stop Simulation : Stop
  wires:
  Relational Operator/1 -> Stop Simulation/1
  SOC/1 -> Relational Operator/1
  Const/1 -> Relational Operator/2

== system advisor_ess_options/energy storage <ess> nnet/Limits ==
  power req : Inport  Port=1  PortWidth=-1  SampleTime=-1
  power  available from battery : Inport  Port=2  PortWidth=-1  SampleTime=-1
  Const{1..4} (4 alike) : Constant  Value=0
  Relational Operator1 : RelationalOperator  Operator===
  limited by battery : Logic  Operator=NOT  Inputs=1
  tag scope: ess_maxV_limited=global, ess_minV_limited=global, ess_pwr_limited=global, ess_soc_limited=global, mc_voltage_limited=global
  wires:
  Const1/1 -> [ess_soc_limited]
  Const2/1 -> [ess_maxV_limited]
  Const3/1 -> [ess_minV_limited]
  Const4/1 -> [mc_voltage_limited]
  power  available from battery/1 -> Relational Operator1/2
  power req/1 -> Relational Operator1/1
  limited by battery/1 -> [ess_pwr_limited]
  Relational Operator1/1 -> limited by battery/1

== system advisor_ess_options/energy storage <ess> nnet/NNet ==
  Preq : Inport  Port=1  PortWidth=-1  SampleTime=-1
  SOC : Inport  Port=2  PortWidth=-1  SampleTime=-1
  Enable : EnablePort
  De-Normalizer1 Voltage : Fcn  Expr=(u-0.2)*(ess_MMo(2,2)-ess_MMo(2,1))/(0.8-0.2)+ess_MMo(2,1)
  De-Normalizer2 Current : Fcn  Expr=(u-0.2)*(ess_MMo(1,2)-ess_MMo(1,1))/(0.8-0.2)+ess_MMo(1,1)
  Demux : Demux  Outputs=2
  Mux : Mux  Inputs=2
  Neural Network : Subsystem
  Normalizer Power : Fcn  Expr=(u-ess_MMi(1,1))/(ess_MMi(1,2)-ess_MMi(1,1))
  Normalizer SOC : Fcn  Expr=(u-ess_MMi(2,1))/(ess_MMi(2,2)-ess_MMi(2,1))
  V : Outport  Port=1  InitialOutput=0
  i : Outport  Port=2  OutputWhenDisabled=reset  InitialOutput=0
  wires:
  Mux/1 -> Neural Network/1("p{1}")
  Neural Network/1("y{1}") -> Demux/1
  Preq/1 -> Normalizer Power/1
  Normalizer Power/1 -> Mux/1
  SOC/1 -> Normalizer SOC/1
  Normalizer SOC/1 -> Mux/2
  De-Normalizer2 Current/1 -> i/1
  Demux/1 -> De-Normalizer2 Current/1
  Demux/2 -> De-Normalizer1 Voltage/1
  De-Normalizer1 Voltage/1 -> V/1

== system advisor_ess_options/energy storage <ess> nnet/No Thermal model ==
  Const1 : Constant  Value=0
  Const2 : Constant  Value=amb_tmp
  Const3 : Constant  Value=0
  To WS1 : ToWorkspace  VariableName=ess_pwr_loss_a  SampleTime=0
  To WS2 : ToWorkspace  VariableName=ess_mod_tmp  SampleTime=0
  To WS3 : ToWorkspace  VariableName=ess_air_tmp  SampleTime=0
  To WS4 : ToWorkspace  VariableName=ess_air_th_pwr  SampleTime=0
  wires:
  Const1/1 -> To WS1/1
  Const2/1 -> To WS2/1, To WS3/1
  Const3/1 -> To WS4/1

== system advisor_ess_options/energy storage <ess> nnet/SOC algorithm ==
  note: SOC=(Max Ah capacity-Ah used)/Max Ah capacity
  (A) : Inport  Port=1  PortWidth=-1  SampleTime=-1
  tmp (C) : Inport  Port=2  PortWidth=-1  SampleTime=-1
  (sec->hrs) : Gain  Gain=1/3600
  0 <= SOC <= 1 : Saturate  UpperLimit=1  LowerLimit=0
  A-h remaining : Sum  Inputs=-+
  Ah used : Integrator  ExternalReset=none  InitialConditionSource=external  InitialCondition=(1-ess_init_soc)*ess_max_ah_cap  LimitOutput=off  UpperSaturationLimit=inf  LowerSaturationLimit=-inf  ShowSaturationPort=off  ShowStatePort=off  AbsoluteTolerance=auto
  Fcn : Fcn  Expr=1/u
  Fcn1 : Fcn  Expr=(1-ess_init_soc)*u
  SOC : Product  Inputs=2
  Switch : Switch  Threshold=0
  adjusted A : Product  Inputs=2
  coul eff : Lookup  InputValues=ess_tmp  OutputValues=ess_coulombic_eff
  max cap : Lookup  InputValues=ess_tmp  OutputValues=ess_max_ah_cap
  SOC1 : Outport  Port=1  InitialOutput=0
  wires:
  (A)/1 -> Switch/2, Switch/1, adjusted A/1
  Switch/1 -> (sec->hrs)/1
  (sec->hrs)/1 -> Ah used/1
  Ah used/1 -> A-h remaining/1
  Fcn/1 -> SOC/2
  SOC/1 -> 0 <= SOC <= 1/1
  A-h remaining/1 -> SOC/1
  0 <= SOC <= 1/1 -> SOC1/1
  tmp (C)/1 -> max cap/1, coul eff/1
  coul eff/1 -> adjusted A/2
  adjusted A/1 -> Switch/3
  max cap/1 -> A-h remaining/2, Fcn/1, Fcn1/1
  Fcn1/1 -> Ah used/2

== system advisor_ess_options/energy storage <ess> nnet/max pack pwr (W) ==
  SOC : Inport  Port=1  PortWidth=-1  SampleTime=-1
  # batteries : Gain  Gain=ess_module_num
  max power : Lookup  InputValues=ess_max_p_soc  OutputValues=ess_max_p
  ess discharge pwr : Outport  Port=1  InitialOutput=0
  wires:
  SOC/1 -> max power/1
  max power/1 -> # batteries/1
  # batteries/1 -> ess discharge pwr/1

== system advisor_ess_options/energy storage <ess> nnet/stop sim ==
  SOC : Inport  Port=1  PortWidth=-1  SampleTime=-1
  Enable : EnablePort
  Const : Constant  Orientation=up  Value=.001
  Relational Operator : RelationalOperator  Operator=<
  Stop Simulation : Stop
  wires:
  Const/1 -> Relational Operator/2
  SOC/1 -> Relational Operator/1
  Relational Operator/1 -> Stop Simulation/1

== system advisor_ess_options/energy storage <ess> fundamental model/Block NOTES ==
  note: Fundamentally based SOC model developed at BYU
      | Files needed:
      | input1.dat
      | input2.dat
      | input3.dat
      | nrel13cs.dll

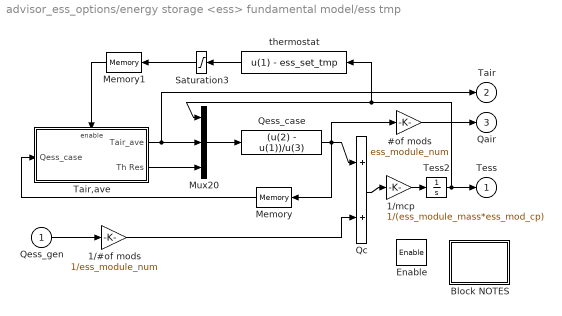
== system advisor_ess_options/energy storage <ess> fundamental model/ess tmp ==
  Qess_gen : Inport  Port=1  PortWidth=-1  SampleTime=-1
  Enable : EnablePort  StatesWhenEnabling=reset
  #of mods : Gain  Gain=ess_module_num
  1/#of mods : Gain  Gain=1/ess_module_num
  1/mcp : Gain  Gain=1/(ess_module_mass*ess_mod_cp)
  Block NOTES : Subsystem
      mask Display: disp('Block\nNOTES')
  Memory : Memory  Orientation=left  X0=cyc_mph(1,2)*.447  InheritSampleTime=off
  Memory1 : Memory  Orientation=left  X0=cyc_mph(1,2)*.447  InheritSampleTime=off
  Mux20 : Mux  Inputs=3
  Qc : Sum  Inputs=++
  Qess_case : Fcn  Expr=(u(2) - u(1))/u(3)
  Saturation3 : Saturate  Orientation=left  UpperLimit=1  LowerLimit=0
  Tair,ave : Subsystem
  Tess2 : Integrator  ExternalReset=none  InitialConditionSource=internal  InitialCondition=ess_mod_init_tmp  LimitOutput=off  UpperSaturationLimit=inf  LowerSaturationLimit=-inf  ShowSaturationPort=off  ShowStatePort=off  AbsoluteTolerance=auto
  thermostat : Fcn  Orientation=left  Expr=u(1) - ess_set_tmp
  Tess : Outport  Port=1  InitialOutput=0
  Tair : Outport  Port=2
  Qair : Outport  Port=3  OutputWhenDisabled=reset  InitialOutput=0
  wires:
  Qc/1 -> 1/mcp/1
  Qess_case/1 -> Qc/1, Memory/1, #of mods/1
  1/mcp/1 -> Tess2/1
  Tess2/1 -> Tess/1, Mux20/1, thermostat/1
  Qess_gen/1 -> 1/#of mods/1
  1/#of mods/1 -> Qc/2
  thermostat/1 -> Saturation3/1
  Saturation3/1 -> Memory1/1
  Memory1/1 -> Tair,ave/Enable
  Memory/1 -> Tair,ave/1(Qess_case)
  #of mods/1 -> Qair/1
  Mux20/1 -> Qess_case/1
  Tair,ave/2(Th Res) -> Mux20/3
  Tair,ave/1(Tair_ave) -> Mux20/2, Tair/1

== system advisor_ess_options/energy storage <ess> fundamental model/max pack pwr (W) ==
  SOC : Inport  Port=1  PortWidth=-1  SampleTime=-1
  # batteries : Gain  Gain=ess_module_num
  max power : Lookup  InputValues=ess_max_p_soc  OutputValues=ess_max_p
  ess discharge pwr : Outport  Port=1  InitialOutput=0
  wires:
  SOC/1 -> max power/1
  max power/1 -> # batteries/1
  # batteries/1 -> ess discharge pwr/1

== system advisor_ess_options/energy storage <ess> fundamental model/stop sim ==
  SOC : Inport  Port=1  PortWidth=-1  SampleTime=-1
  Enable : EnablePort
  Const : Constant  Orientation=up  Value=0.1
  Relational Operator : RelationalOperator  Operator=<
  Stop Simulation : Stop
  wires:
  Const/1 -> Relational Operator/2
  SOC/1 -> Relational Operator/1
  Relational Operator/1 -> Stop Simulation/1

== system advisor_ess_options/energy storage <ess> optima fundamental model/Block NOTES ==
  note: Fundamentally based SOC model developed at BYU
      | Files needed:
      | input1.dat
      | input2.dat
      | input3.dat
      | nrel13cs.dll

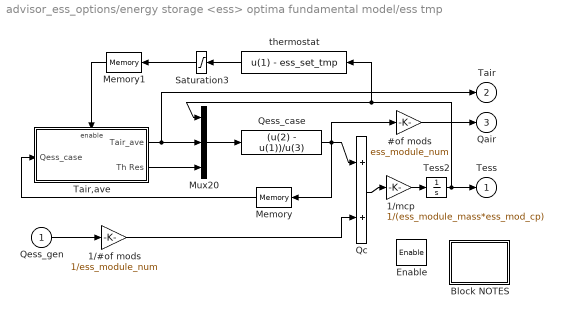
== system advisor_ess_options/energy storage <ess> optima fundamental model/ess tmp ==
  Qess_gen : Inport  Port=1  PortWidth=-1  SampleTime=-1
  Enable : EnablePort  StatesWhenEnabling=reset
  #of mods : Gain  Gain=ess_module_num
  1/#of mods : Gain  Gain=1/ess_module_num
  1/mcp : Gain  Gain=1/(ess_module_mass*ess_mod_cp)
  Block NOTES : Subsystem
      mask Display: disp('Block\nNOTES')
  Memory : Memory  Orientation=left  X0=cyc_mph(1,2)*.447  InheritSampleTime=off
  Memory1 : Memory  Orientation=left  X0=cyc_mph(1,2)*.447  InheritSampleTime=off
  Mux20 : Mux  Inputs=3
  Qc : Sum  Inputs=++
  Qess_case : Fcn  Expr=(u(2) - u(1))/u(3)
  Saturation3 : Saturate  Orientation=left  UpperLimit=1  LowerLimit=0
  Tair,ave : Subsystem
  Tess2 : Integrator  ExternalReset=none  InitialConditionSource=internal  InitialCondition=ess_mod_init_tmp  LimitOutput=off  UpperSaturationLimit=inf  LowerSaturationLimit=-inf  ShowSaturationPort=off  ShowStatePort=off  AbsoluteTolerance=auto
  thermostat : Fcn  Orientation=left  Expr=u(1) - ess_set_tmp
  Tess : Outport  Port=1  InitialOutput=0
  Tair : Outport  Port=2
  Qair : Outport  Port=3  OutputWhenDisabled=reset  InitialOutput=0
  wires:
  Qc/1 -> 1/mcp/1
  Qess_case/1 -> Qc/1, Memory/1, #of mods/1
  1/mcp/1 -> Tess2/1
  Tess2/1 -> Tess/1, Mux20/1, thermostat/1
  Qess_gen/1 -> 1/#of mods/1
  1/#of mods/1 -> Qc/2
  thermostat/1 -> Saturation3/1
  Saturation3/1 -> Memory1/1
  Memory1/1 -> Tair,ave/Enable
  Memory/1 -> Tair,ave/1(Qess_case)
  #of mods/1 -> Qair/1
  Mux20/1 -> Qess_case/1
  Tair,ave/2(Th Res) -> Mux20/3
  Tair,ave/1(Tair_ave) -> Mux20/2, Tair/1

== system advisor_ess_options/energy storage <ess> optima fundamental model/max pack pwr (W) ==
  SOC : Inport  Port=1  PortWidth=-1  SampleTime=-1
  # batteries : Gain  Gain=ess_module_num
  max power : Lookup  InputValues=ess_max_p_soc  OutputValues=ess_max_p
  ess discharge pwr : Outport  Port=1  InitialOutput=0
  wires:
  SOC/1 -> max power/1
  max power/1 -> # batteries/1
  # batteries/1 -> ess discharge pwr/1

== system advisor_ess_options/energy storage <ess> optima fundamental model/stop sim ==
  SOC : Inport  Port=1  PortWidth=-1  SampleTime=-1
  Enable : EnablePort
  Const : Constant  Orientation=up  Value=.001
  Relational Operator : RelationalOperator  Operator=<
  Stop Simulation : Stop
  wires:
  Const/1 -> Relational Operator/2
  SOC/1 -> Relational Operator/1
  Relational Operator/1 -> Stop Simulation/1

== system advisor_ess_options/energy storage <ess>/ess tmp/Block NOTES ==
  note: This block models the thermal behavior of a battery module with active air cooling.
      | The module is modeled as a single lumped thermal mass.
      | The fan is on whenever the battery temp is > the set temp.

== system advisor_ess_options/energy storage <ess>/ess tmp/Tair,ave ==
  Qess_case : Inport  Port=1  PortWidth=-1  SampleTime=-1
  Enable : EnablePort  StatesWhenEnabling=reset
  Block NOTES : Subsystem
      mask Display: disp('Block\nNOTES')
  Tamb-(Q/mcp)/2 : Fcn  Expr=amb_tmp - (u(1)/(ess_mod_airflow*air_cp))/2
  do ex calcs?1 : Constant  Value=ess_th_res_on
  Tair_ave : Outport  Port=1  OutputWhenDisabled=reset  InitialOutput=amb_tmp
  Th Res : Outport  Port=2  OutputWhenDisabled=reset  InitialOutput=ess_th_res_off
  wires:
  do ex calcs?1/1 -> Th Res/1
  Qess_case/1 -> Tamb-(Q/mcp)/2/1
  Tamb-(Q/mcp)/2/1 -> Tair_ave/1

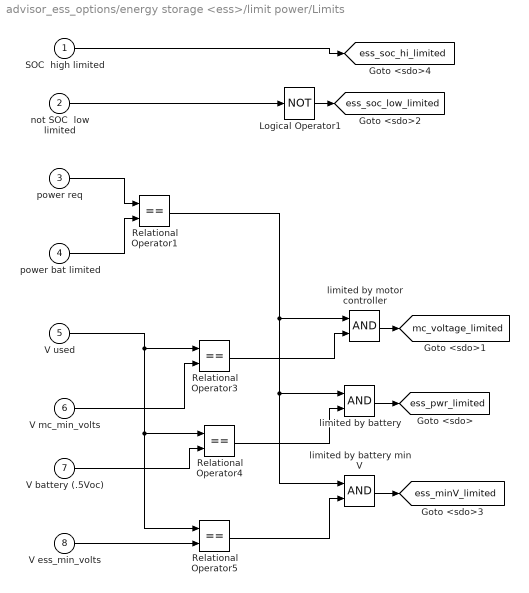
== system advisor_ess_options/energy storage <ess>/limit power/Limits ==
  SOC  high limited : Inport  Port=1  PortWidth=-1  SampleTime=-1
  not SOC  low limited : Inport  Port=2  PortWidth=-1  SampleTime=-1
  power req : Inport  Port=3  PortWidth=-1  SampleTime=-1
  power bat limited : Inport  Port=4  PortWidth=-1  SampleTime=-1
  V used : Inport  Port=5  PortWidth=-1  SampleTime=-1
  V mc_min_volts : Inport  Port=6  PortWidth=-1  SampleTime=-1
  V battery (.5Voc) : Inport  Port=7  PortWidth=-1  SampleTime=-1
  V ess_min_volts : Inport  Port=8  PortWidth=-1  SampleTime=-1
  Logical Operator1 : Logic  Operator=NOT  Inputs=1
  Relational Operator{1,3..5} (4 alike) : RelationalOperator  Operator===
  limited by battery : Logic  Operator=AND  Inputs=2
  limited by battery min V : Logic  Operator=AND  Inputs=2
  limited by motor controller : Logic  Operator=AND  Inputs=2
  tag scope: ess_minV_limited=global, ess_pwr_limited=global, ess_soc_hi_limited=global, ess_soc_low_limited=global, mc_voltage_limited=global
  wires:
  SOC  high limited/1 -> [ess_soc_hi_limited]
  not SOC  low limited/1 -> Logical Operator1/1
  Logical Operator1/1 -> [ess_soc_low_limited]
  power req/1 -> Relational Operator1/1
  Relational Operator5/1 -> limited by battery min V/2
  Relational Operator4/1 -> limited by battery/2
  Relational Operator1/1 -> limited by battery min V/1, limited by battery/1, limited by motor controller/1
  Relational Operator3/1 -> limited by motor controller/2
  limited by battery min V/1 -> [ess_minV_limited]
  limited by battery/1 -> [ess_pwr_limited]
  limited by motor controller/1 -> [mc_voltage_limited]
  V ess_min_volts/1 -> Relational Operator5/2
  V battery (.5Voc)/1 -> Relational Operator4/2
  V used/1 -> Relational Operator5/1, Relational Operator4/1, Relational Operator3/1
  V mc_min_volts/1 -> Relational Operator3/2
  power bat limited/1 -> Relational Operator1/2

== system advisor_ess_options/energy storage <ess>/max pack pwr (W)1/Rdis (ohms) ==
  x0 : Inport  Port=1  PortWidth=-1  SampleTime=-1
  y0 : Inport  Port=2  PortWidth=-1  SampleTime=-1
  Mux : Mux  Inputs=2
  S-function : S-Function  FunctionName=sftable2  Parameters=xindex, yindex, table  PortCounts=[]  SFunctionModules=''
  table out : Outport  Port=1  InitialOutput=0
  wires:
  y0/1 -> Mux/2
  S-function/1 -> table out/1
  x0/1 -> Mux/1
  Mux/1 -> S-function/1

== system advisor_ess_options/energy storage <ess>/max pack pwr (W)1/VOC (V) ==
  x0 : Inport  Port=1  PortWidth=-1  SampleTime=-1
  y0 : Inport  Port=2  PortWidth=-1  SampleTime=-1
  Mux : Mux  Inputs=2
  S-function : S-Function  FunctionName=sftable2  Parameters=xindex, yindex, table  PortCounts=[]  SFunctionModules=''
  table out : Outport  Port=1  InitialOutput=0
  wires:
  y0/1 -> Mux/2
  S-function/1 -> table out/1
  x0/1 -> Mux/1
  Mux/1 -> S-function/1

== system advisor_ess_options/energy storage <ess>/pack Voc, Rint/Rchg (ohms) ==
  x0 : Inport  Port=1  PortWidth=-1  SampleTime=-1
  y0 : Inport  Port=2  PortWidth=-1  SampleTime=-1
  Mux : Mux  Inputs=2
  S-function : S-Function  FunctionName=sftable2  Parameters=xindex, yindex, table  PortCounts=[]  SFunctionModules=''
  table out : Outport  Port=1  InitialOutput=0
  wires:
  Mux/1 -> S-function/1
  x0/1 -> Mux/1
  S-function/1 -> table out/1
  y0/1 -> Mux/2

== system advisor_ess_options/energy storage <ess>/pack Voc, Rint/Rdis (ohms) ==
  x0 : Inport  Port=1  PortWidth=-1  SampleTime=-1
  y0 : Inport  Port=2  PortWidth=-1  SampleTime=-1
  Mux : Mux  Inputs=2
  S-function : S-Function  FunctionName=sftable2  Parameters=xindex, yindex, table  PortCounts=[]  SFunctionModules=''
  table out : Outport  Port=1  InitialOutput=0
  wires:
  Mux/1 -> S-function/1
  x0/1 -> Mux/1
  S-function/1 -> table out/1
  y0/1 -> Mux/2

== system advisor_ess_options/energy storage <ess>/pack Voc, Rint/VOC (V) ==
  x0 : Inport  Port=1  PortWidth=-1  SampleTime=-1
  y0 : Inport  Port=2  PortWidth=-1  SampleTime=-1
  Mux : Mux  Inputs=2
  S-function : S-Function  FunctionName=sftable2  Parameters=xindex, yindex, table  PortCounts=[]  SFunctionModules=''
  table out : Outport  Port=1  InitialOutput=0
  wires:
  Mux/1 -> S-function/1
  x0/1 -> Mux/1
  S-function/1 -> table out/1
  y0/1 -> Mux/2

== system advisor_ess_options/energy storage <ess> nnet/NNet/Neural Network ==
  "p{1}" : Inport  Port=1  PortWidth=2  SampleTime=-1
  Layer 1 : Subsystem
  Layer 2 : Subsystem
  "y{1}" : Outport  Port=1  InitialOutput=[0;0]
  wires:
  "p{1}"/1 -> Layer 1/1("p{1}")
  Layer 1/1("a{1}") -> [feedback1]
  [feedback1] -> Layer 2/1("a{1} ")
  Layer 2/1("a{2}") -> "y{1}"/1

== system advisor_ess_options/energy storage <ess> fundamental model/ess tmp/Block NOTES ==
  note: This block models the thermal behavior of a battery module with active air cooling.
      | The module is modeled as a single lumped thermal mass.
      | The fan is on whenever the battery temp is > the set temp.

== system advisor_ess_options/energy storage <ess> fundamental model/ess tmp/Tair,ave ==
  Qess_case : Inport  Port=1  PortWidth=-1  SampleTime=-1
  Enable : EnablePort  StatesWhenEnabling=reset
  Block NOTES : Subsystem
      mask Display: disp('Block\nNOTES')
  Tamb-(Q/mcp)/2 : Fcn  Expr=amb_tmp - (u(1)/(ess_mod_airflow*air_cp))/2
  do ex calcs?1 : Constant  Value=ess_th_res_on
  Tair_ave : Outport  Port=1  OutputWhenDisabled=reset  InitialOutput=amb_tmp
  Th Res : Outport  Port=2  OutputWhenDisabled=reset  InitialOutput=ess_th_res_off
  wires:
  Tamb-(Q/mcp)/2/1 -> Tair_ave/1
  Qess_case/1 -> Tamb-(Q/mcp)/2/1
  do ex calcs?1/1 -> Th Res/1

== system advisor_ess_options/energy storage <ess> optima fundamental model/ess tmp/Block NOTES ==
  note: This block models the thermal behavior of a battery module with active air cooling.
      | The module is modeled as a single lumped thermal mass.
      | The fan is on whenever the battery temp is > the set temp.

== system advisor_ess_options/energy storage <ess> optima fundamental model/ess tmp/Tair,ave ==
  Qess_case : Inport  Port=1  PortWidth=-1  SampleTime=-1
  Enable : EnablePort  StatesWhenEnabling=reset
  Block NOTES : Subsystem
      mask Display: disp('Block\nNOTES')
  Tamb-(Q/mcp)/2 : Fcn  Expr=amb_tmp - (u(1)/(ess_mod_airflow*air_cp))/2
  do ex calcs?1 : Constant  Value=ess_th_res_on
  Tair_ave : Outport  Port=1  OutputWhenDisabled=reset  InitialOutput=amb_tmp
  Th Res : Outport  Port=2  OutputWhenDisabled=reset  InitialOutput=ess_th_res_off
  wires:
  Tamb-(Q/mcp)/2/1 -> Tair_ave/1
  Qess_case/1 -> Tamb-(Q/mcp)/2/1
  do ex calcs?1/1 -> Th Res/1

== system advisor_ess_options/energy storage <ess>/ess tmp/Tair,ave/Block NOTES ==
  note: This block determins the average temperature of the cooling air over the module.

== system advisor_ess_options/energy storage <ess> nnet/NNet/Neural Network/Layer 1 ==
  "p{1}" : Inport  Port=1  PortWidth=2  SampleTime=-1
  Delays 1 : Subsystem
      mask Display: disp('TDL')
  "IW{1,1}" : Subsystem
      mask Display: disp('weight')
  "b{1}" : Constant  Value=[-6.0348629999999996;2.0410720000000002;2.002373]
      mask Display: disp('bias')
  logsig : Subsystem
      mask Display: plot([-1 1],[0 0],[-1 -.9 -.8 -.7 -.6 -.5 -.4 -.3 -.2 -.1 0 .1 .2 .3 .4 .5 .6 .7 .8 .9 1],1./(1+exp(-8*[-1 -.9 -.8 -.7 -.6 -.5 -.4 -.3 -.2 -.1 0 .1 .2 .3 .4 .5 .6 .7 .8 .9 1]))+.01)
  netsum : Sum  Inputs=2
      mask Display: disp('+')
  "a{1}" : Outport  Port=1  InitialOutput=[0;0;0]
  wires:
  "p{1}"/1 -> Delays 1/1("p{1}")
  Delays 1/1("pd{1,1}") -> "IW{1,1}"/1("pd{1,1}")
  "IW{1,1}"/1("iz{1,1}") -> netsum/1
  "b{1}"/1 -> netsum/2
  netsum/1 -> logsig/1(n)
  logsig/1(a) -> "a{1}"/1

== system advisor_ess_options/energy storage <ess> nnet/NNet/Neural Network/Layer 2 ==
  "a{1} " : Inport  Port=1  PortWidth=3  SampleTime=-1
  Delays 1 : Subsystem
      mask Display: disp('TDL')
  "LW{2,1}" : Subsystem
      mask Display: disp('weight')
  "b{2}" : Constant  Value=[3.0652170000000001;-2.2814760000000001]
      mask Display: disp('bias')
  logsig : Subsystem
      mask Display: plot([-1 1],[0 0],[-1 -.9 -.8 -.7 -.6 -.5 -.4 -.3 -.2 -.1 0 .1 .2 .3 .4 .5 .6 .7 .8 .9 1],1./(1+exp(-8*[-1 -.9 -.8 -.7 -.6 -.5 -.4 -.3 -.2 -.1 0 .1 .2 .3 .4 .5 .6 .7 .8 .9 1]))+.01)
  netsum : Sum  Inputs=2
      mask Display: disp('+')
  "a{2}" : Outport  Port=1  InitialOutput=[0;0]
  wires:
  "a{1} "/1 -> Delays 1/1("p{2}")
  Delays 1/1("pd{2,1}") -> "LW{2,1}"/1("ad{2,1}")
  "LW{2,1}"/1("lz{2,1}") -> netsum/1
  "b{2}"/1 -> netsum/2
  netsum/1 -> logsig/1(n)
  logsig/1(a) -> "a{2}"/1

== system advisor_ess_options/energy storage <ess> fundamental model/ess tmp/Tair,ave/Block NOTES ==
  note: This block determins the average temperature of the cooling air over the module.

== system advisor_ess_options/energy storage <ess> optima fundamental model/ess tmp/Tair,ave/Block NOTES ==
  note: This block determins the average temperature of the cooling air over the module.

== system advisor_ess_options/energy storage <ess> nnet/NNet/Neural Network/Layer 1/Delays 1 ==
  "p{1}" : Inport  Orientation=down  Port=1  PortWidth=2  SampleTime=-1
  mux : Mux  Inputs=1
  "pd{1,1}" : Outport  Port=1  InitialOutput=0
  wires:
  "p{1}"/1 -> mux/1
  mux/1 -> "pd{1,1}"/1

== system advisor_ess_options/energy storage <ess> nnet/NNet/Neural Network/Layer 1/IW{1,1} ==
  "pd{1,1}" : Inport  Port=1  PortWidth=2  SampleTime=-1
  "IW{1,1}(1,:)'" : Constant  Value=[-4.5598890000000001;5.793647]
      mask Display: disp('weights')
  "IW{1,1}(2,:)'" : Constant  Value=[-2.8283469999999999;1.417519]
      mask Display: disp('weights')
  "IW{1,1}(3,:)'" : Constant  Value=[-2.3043559999999998;-1.4467429999999999]
      mask Display: disp('weights')
  Mux : Mux  Inputs=3
  dotprod1 : Subsystem
  dotprod2 : Subsystem
  dotprod3 : Subsystem
  "iz{1,1}" : Outport  Port=1  InitialOutput=0
  wires:
  "IW{1,1}(1,:)'"/1 -> dotprod1/1(w)
  dotprod1/1(z) -> Mux/1
  "IW{1,1}(2,:)'"/1 -> dotprod2/1(w)
  "pd{1,1}"/1 -> dotprod1/2(p), dotprod2/2(p), dotprod3/2(p)
  dotprod2/1(z) -> Mux/2
  "IW{1,1}(3,:)'"/1 -> dotprod3/1(w)
  dotprod3/1(z) -> Mux/3
  Mux/1 -> "iz{1,1}"/1

== system advisor_ess_options/energy storage <ess> nnet/NNet/Neural Network/Layer 1/logsig ==
  n : Inport  Port=1  PortWidth=-1  SampleTime=-1
  Exp : ElementaryMath  Operator=exp
  Gain : Gain  Gain=-1
  Reciprocal : ElementaryMath  Operator=reciprocal
  Sum : Sum  Inputs=++
  one : Constant  Value=1
  a : Outport  Port=1  InitialOutput=0
  wires:
  Reciprocal/1 -> a/1
  Sum/1 -> Reciprocal/1
  one/1 -> Sum/2
  Exp/1 -> Sum/1
  Gain/1 -> Exp/1
  n/1 -> Gain/1

== system advisor_ess_options/energy storage <ess> nnet/NNet/Neural Network/Layer 2/Delays 1 ==
  "p{2}" : Inport  Orientation=down  Port=1  PortWidth=3  SampleTime=-1
  mux : Mux  Inputs=1
  "pd{2,1}" : Outport  Port=1  InitialOutput=0
  wires:
  "p{2}"/1 -> mux/1
  mux/1 -> "pd{2,1}"/1
